simulink model "sim12ex3"  (Simulink 2.09)
settings: Solver=ode45  StartTime=0.0  StopTime=10  MaxStep=.1  RelTol=1e-3  AbsTol=1e-3
settings Model: SaveTime=off  SaveOutput=off  ConsistencyChecking=off  RTWTemplateMakefile=grt_vc.tmf

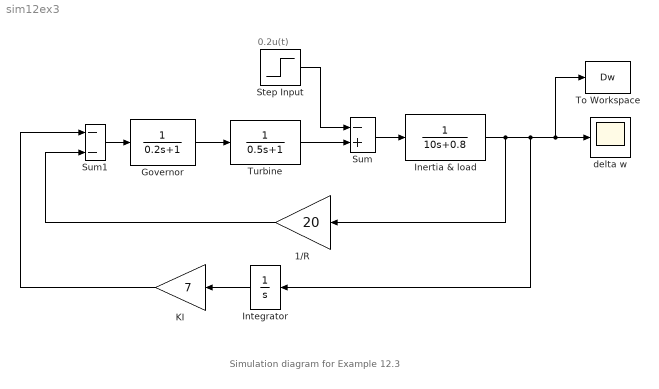
== system sim12ex3 ==
  note: 0.2u(t)
  note: Simulation diagram for Example 12.3
  1/R : Gain  Orientation=left  Gain=20
  Governor : TransferFcn  Numerator=[1]  Denominator="[0.2   1]"
  Inertia & load : TransferFcn  Numerator=[1]  Denominator="[10  0.8]"
  Integrator : Integrator  Orientation=left  ExternalReset=none  InitialConditionSource=internal  InitialCondition=0  LimitOutput=off  UpperSaturationLimit=inf  LowerSaturationLimit=-inf  ShowSaturationPort=off  ShowStatePort=off  AbsoluteTolerance=auto
  KI : Gain  Orientation=left  Gain=7
  Step Input : Step  Time=100  Before=0.2  After=.2
  Sum : Sum  Inputs=-+
  Sum1 : Sum  Inputs=--
  To Workspace : ToWorkspace  VariableName=Dw  SampleTime=0
      settings: Buffer=1000
  Turbine : TransferFcn  Numerator=[1]  Denominator="[0.5  1]"
  delta w : Scope
      settings: TickLabels=on  TimeRange=auto  YMin=-5  YMax=5  SaveToWorkspace=off  SaveName=ScopeData
  wires:
  Governor/1 -> Turbine/1
  Turbine/1 -> Sum/2
  Sum/1 -> Inertia & load/1
  Sum1/1 -> Governor/1
  Integrator/1 -> KI/1
  KI/1 -> Sum1/1
  1/R/1 -> Sum1/2
  Step Input/1 -> Sum/1
  Inertia & load/1 -> 1/R/1, Integrator/1, delta w/1, To Workspace/1
